simulink model "LKAS_AutoSave_DF_20211126_SW5"  (R2018b)
settings: Solver=FixedStepDiscrete  StartTime=0.0  StopTime=10.0  FixedStep=0.01  RelTol=1e-3
undefined symbols (not defined in the file): LKA_CarWidth, LKA_SampleTime, LKA_StrRatio_C, LKA_Veh2CamL_C, LKA_Veh2CamW_C, LKA_WhlBaseL_C, LL_CompSWA_C, LL_CrvtPrvwT_C, LL_DesDvt_C, LL_DvtComp_C, LL_DvtPrvwT_C, LL_DvtSpdDet_vDvtSpdMin_C, LL_HdAgExT_C, LL_HdAgPrvwT_C, LL_LAccMax_C, LL_LAccRMax_C, LL_LDW_EarliestWarnLine_C, LL_LDW_LatestWarnLine_C, LL_LDWS_SUPPRESS_HEADING, LL_LFClb_TFC_FfCtlRatio_C, LL_LFClb_TFC_KdBalance_C, LL_LFClb_TFC_KdMaxSWA_C, LL_LFClb_TFC_KdV1_C, LL_LFClb_TFC_KdV2_C, LL_LFClb_TFC_KdVehSpdLwr_C, LL_LFClb_TFC_KdVehSpdUpr_C, LL_LFClb_TFC_Ki_C, LL_LFClb_TFC_KiMaxSWA_C, LL_LFClb_TFC_Kp_C, LL_LFClb_TFC_KpKlat_C, LL_LFClb_TFC_KpV1_C, LL_LFClb_TFC_KpV2_C, LL_LFClb_TFC_KpVehSpdLwr_C, LL_LFClb_TFC_KpVehSpdUpr_C, LL_LFClb_TFC_PrvwT_C, LL_LKA_EarliestWarnLine_C, LL_LKA_LatestWarnLine_C, LL_LKAExPrcs_ExitC0Dvt, LL_LKAExPrcs_ExitC0Swt, LL_LKAExPrcs_tiExitTime1, LL_LKAExPrcs_tiExitTime2, LL_LKAExPrcs_tiExitTime3, LL_LKAS_OUT_OF_CONTROL_LAT_VEL, LL_LKAS_OUT_OF_CONTROL_TTLC, LL_LKASWASyn_M0, LL_LKASWASyn_M1, LL_LKASWASyn_M2, LL_LKASWASyn_M3K, LL_LKASWASyn_SWAaddMax, LL_LKASWASyn_T2, LL_LKASWASyn_tiTrqSwaRtTime, LL_LKASWASyn_tiTrqSwaTime, LL_LKASWASyn_TrqMax, LL_LKASWASyn_TrqSwaAddSwt, LL_LKASWASyn_TrqSwaRateDiff, LL_LSpdCompT_C, LL_lStpLngth_C, LL_MAX_DELAY_EPSSTAR_TIME, LL_MAX_DRIVER_TORQUE_DISABLE, LL_MAX_DRIVER_TORQUE_ENABLE ... (+38)
libraries: simulink x137, canmsglib x10, dspstat3 x3, simulink_extras x1
(part 11 of 13)

== system LKAS_AutoSave_DF_20211126_SW5/LKAS/LL/LLOn/LL State Determination (LLStateDet)/LL State Machine Conditions (LLSMCon)/Disable Condition (DisblC)/LKA Own Condition (LKAOwnC)/LKA Own Condition Synthesis (LKAOwnCSyn) ==
  LKAOwnCSyn_stDACMode : Inport
  LKAOwnCSyn_stVehLSpdC : Inport  Port=2
  LKAOwnCSyn_stVehPosChk : Inport  Port=3
  LKAOwnCSyn_stEPSCtlEC : Inport  Port=4
  Compare To Constant : simulink/Logic and Bit Operations/Compare To Constant  relop===  const=2  OutDataTypeStr=boolean
  Compare To Constant1 : simulink/Logic and Bit Operations/Compare To Constant  relop===  const=1  OutDataTypeStr=boolean
  Compare To Constant2 : simulink/Logic and Bit Operations/Compare To Constant  relop===  const=1  OutDataTypeStr=boolean
  Compare To Constant3 : simulink/Logic and Bit Operations/Compare To Constant  relop===  const=1  OutDataTypeStr=boolean
  Logical Operator : Logic  AllPortsSameDT=off  OutDataTypeStr=boolean
  Logical Operator1 : Logic  Operator=OR  Inputs=3  AllPortsSameDT=off  OutDataTypeStr=boolean
  LKAOwnCSyn_stLKAOwnCSyn : Outport
  wires:
  Compare To Constant3/1 -> Logical Operator1/1
  LKAOwnCSyn_stVehLSpdC/1 -> Compare To Constant3/1
  Logical Operator1/1 -> Logical Operator/2
  Compare To Constant/1 -> Logical Operator/1
  Compare To Constant1/1 -> Logical Operator1/2
  Compare To Constant2/1 -> Logical Operator1/3
  LKAOwnCSyn_stEPSCtlEC/1 -> Compare To Constant2/1
  Logical Operator/1 -> LKAOwnCSyn_stLKAOwnCSyn/1
  LKAOwnCSyn_stVehPosChk/1 -> Compare To Constant1/1
  LKAOwnCSyn_stDACMode/1 -> Compare To Constant/1

== system LKAS_AutoSave_DF_20211126_SW5/LKAS/LL/LLOn/LL State Determination (LLStateDet)/LL State Machine Conditions (LLSMCon)/Disable Condition (DisblC)/LKA Own Condition (LKAOwnC)/Vehicle Lateral Speed Condition (VehLSpdC) ==
  VehLSpdC_bsTTLC : Inport
  VehLSpdC_vVehLSpdMax_C : Inport  Port=2
  Abs : Abs
  Abs1 : Abs
  Bus Selector : BusSelector  OutputSignals=vLft,vRgt
  Logical Operator : Logic  Operator=OR  AllPortsSameDT=off  OutDataTypeStr=boolean
  Relational Operator1 : RelationalOperator  OutDataTypeStr=boolean  RndMeth=Nearest
  Relational Operator2 : RelationalOperator  OutDataTypeStr=boolean  RndMeth=Nearest
  VehLSpdC_stVehLSpdC : Outport
  wires:
  Logical Operator/1 -> VehLSpdC_stVehLSpdC/1
  Relational Operator2/1 -> Logical Operator/2
  Relational Operator1/1 -> Logical Operator/1
  VehLSpdC_vVehLSpdMax_C/1 -> Relational Operator1/2, Relational Operator2/2
  Abs1/1 -> Relational Operator2/1
  Bus Selector/2 -> Abs1/1  "<vRgt>"
  Bus Selector/1 -> Abs/1  "<vLft>"
  Abs/1 -> Relational Operator1/1
  VehLSpdC_bsTTLC/1 -> Bus Selector/1

== system LKAS_AutoSave_DF_20211126_SW5/LKAS/LL/LLOn/LL State Determination (LLStateDet)/LL State Machine Conditions (LLSMCon)/Disable Condition (DisblC)/LKA Own Condition (LKAOwnC)/Vehicle Position Check (VehPosChk) ==
  VehPosChk_lLftDvt : Inport
  VehPosChk_lRgtDvt : Inport  Port=2
  VehPosChk_lAlrmLine_C : Inport  Port=3
  Logical Operator : Logic  Operator=OR  AllPortsSameDT=off  OutDataTypeStr=boolean
  Relational Operator1 : RelationalOperator  Operator=<=  OutDataTypeStr=boolean  RndMeth=Nearest
  Relational Operator2 : RelationalOperator  Operator=<=  OutDataTypeStr=boolean  RndMeth=Nearest
  VehPosChk_stVehPosChk : Outport
  wires:
  VehPosChk_lRgtDvt/1 -> Relational Operator2/1
  VehPosChk_lLftDvt/1 -> Relational Operator1/1
  Logical Operator/1 -> VehPosChk_stVehPosChk/1
  Relational Operator2/1 -> Logical Operator/2
  Relational Operator1/1 -> Logical Operator/1
  VehPosChk_lAlrmLine_C/1 -> Relational Operator2/2, Relational Operator1/2

== system LKAS_AutoSave_DF_20211126_SW5/LKAS/LL/LLOn/LL State Determination (LLStateDet)/LL State Machine Conditions (LLSMCon)/Disable Condition (DisblC)/Lane Condition (LaneC)/Lane C1 Detection (LaneC1Det) ==
  LaneWDet_facmL0C1 : Inport
  LaneWDet_facmR0C1 : Inport  Port=2
  Abs : Abs
  Add : Sum  Inputs=+-  OutDataTypeStr=single
  Compare To Constant1 : simulink/Logic and Bit Operations/Compare To Constant  relop=>  const=0.040  OutDataTypeStr=boolean
  LaneC1Det_stLaneC1DetFlg : Outport
  wires:
  Abs/1 -> Compare To Constant1/1
  Compare To Constant1/1 -> LaneC1Det_stLaneC1DetFlg/1
  Add/1 -> Abs/1
  LaneWDet_facmL0C1/1 -> Add/1
  LaneWDet_facmR0C1/1 -> Add/2

== system LKAS_AutoSave_DF_20211126_SW5/LKAS/LL/LLOn/LL State Determination (LLStateDet)/LL State Machine Conditions (LLSMCon)/Disable Condition (DisblC)/Lane Condition (LaneC)/Lane Condition Synthesis (LaneCSyn) ==
  LaneCSyn_stLaneQlECFlg : Inport
  LaneCSyn_stLaneWDetFlg : Inport  Port=2
  LaneCSyn_stLaneCrvtDetFlg : Inport  Port=3
  LaneCSyn_stLaneC1DetFlg : Inport  Port=4
  Logical Operator3 : Logic  Operator=OR  Inputs=4  AllPortsSameDT=off  OutDataTypeStr=boolean
  LaneCSyn_stLaneCSyn : Outport
  wires:
  LaneCSyn_stLaneC1DetFlg/1 -> Logical Operator3/4
  LaneCSyn_stLaneWDetFlg/1 -> Logical Operator3/2
  Logical Operator3/1 -> LaneCSyn_stLaneCSyn/1
  LaneCSyn_stLaneCrvtDetFlg/1 -> Logical Operator3/3
  LaneCSyn_stLaneQlECFlg/1 -> Logical Operator3/1

== system LKAS_AutoSave_DF_20211126_SW5/LKAS/LL/LLOn/LL State Determination (LLStateDet)/LL State Machine Conditions (LLSMCon)/Disable Condition (DisblC)/Lane Condition (LaneC)/Lane Curvature Detection (LaneCrvtDet) ==
  LaneCrvtDet_crPrvwCrvt : Inport
  LaneCrvtDet_crLaneCrvtMax_C : Inport  Port=2
  Abs : Abs
  Constant : Constant  Value=0  OutDataTypeStr=single  SampleTime=-1
  Interval Test Dynamic : simulink/Logic and Bit Operations/Interval Test Dynamic  IntervalClosedRight=on  IntervalClosedLeft=on  OutDataTypeStr=boolean
      settings: SourceProductName=Simulink  SourceProductBaseCode=SL
  Logical Operator : Logic  Operator=NOT  AllPortsSameDT=off  OutDataTypeStr=boolean
  LaneCrvtDet_stLaneCrvtDetFlg : Outport
  wires:
  Abs/1 -> Interval Test Dynamic/2
  LaneCrvtDet_crPrvwCrvt/1 -> Abs/1
  Constant/1 -> Interval Test Dynamic/3
  LaneCrvtDet_crLaneCrvtMax_C/1 -> Interval Test Dynamic/1
  Logical Operator/1 -> LaneCrvtDet_stLaneCrvtDetFlg/1
  Interval Test Dynamic/1 -> Logical Operator/1

== system LKAS_AutoSave_DF_20211126_SW5/LKAS/LL/LLOn/LL State Determination (LLStateDet)/LL State Machine Conditions (LLSMCon)/Disable Condition (DisblC)/Lane Condition (LaneC)/Lane Quality Disable Condition (LaneQlDC) ==
  LaneQlDC_stFacmL0Ql : Inport
  LaneQlDC_stFacmR0Ql : Inport  Port=2
  Compare To Constant : simulink/Logic and Bit Operations/Compare To Constant  relop=<  const=3  OutDataTypeStr=boolean
  Compare To Constant1 : simulink/Logic and Bit Operations/Compare To Constant  relop=<  const=3  OutDataTypeStr=boolean
  Logical Operator : Logic  AllPortsSameDT=off  OutDataTypeStr=boolean
  LaneQlDC_stLaneQlDCFlg : Outport
  wires:
  Logical Operator/1 -> LaneQlDC_stLaneQlDCFlg/1
  Compare To Constant1/1 -> Logical Operator/2
  Compare To Constant/1 -> Logical Operator/1
  LaneQlDC_stFacmR0Ql/1 -> Compare To Constant1/1
  LaneQlDC_stFacmL0Ql/1 -> Compare To Constant/1

== system LKAS_AutoSave_DF_20211126_SW5/LKAS/LL/LLOn/LL State Determination (LLStateDet)/LL State Machine Conditions (LLSMCon)/Disable Condition (DisblC)/Lane Condition (LaneC)/Lane Width Detection (LaneWDet) ==
  LaneWDet_LaneWidth : Inport
  LaneWDet_lLaneWMax : Inport  Port=2
  LaneWDet_lLaneWMin : Inport  Port=3
  Abs1 : Abs
  Compare To Zero : simulink/Logic and Bit Operations/Compare To Zero  relop===  OutDataTypeStr=boolean
  Interval Test Dynamic : simulink/Logic and Bit Operations/Interval Test Dynamic  IntervalClosedRight=on  IntervalClosedLeft=on  OutDataTypeStr=boolean
      settings: SourceProductName=Simulink  SourceProductBaseCode=SL
  LaneWDet_stLaneWDetFlg : Outport
  wires:
  LaneWDet_LaneWidth/1 -> Abs1/1
  Abs1/1 -> Interval Test Dynamic/2
  LaneWDet_lLaneWMin/1 -> Interval Test Dynamic/3
  LaneWDet_lLaneWMax/1 -> Interval Test Dynamic/1
  Compare To Zero/1 -> LaneWDet_stLaneWDetFlg/1
  Interval Test Dynamic/1 -> Compare To Zero/1

== system LKAS_AutoSave_DF_20211126_SW5/LKAS/LL/LLOn/LL State Determination (LLStateDet)/LL State Machine Conditions (LLSMCon)/Disable Condition (DisblC)/Subsystem/Subsystem ==
  in1 : Inport
  Add : Sum
  Cast To Single : DataTypeConversion  OutDataTypeStr=uint8
  Memory : Memory  InheritSampleTime=on
  Saturation : Saturate  UpperLimit=1  LowerLimit=0
      settings: AttributesFormatString="Min = %<LowerLimit>  Max = %<UpperLimit>"
  Out1 : Outport
  wires:
  Saturation/1 -> Out1/1, Add/2
  Add/1 -> Memory/1
  Memory/1 -> Saturation/1
  in1/1 -> Cast To Single/1
  Cast To Single/1 -> Add/1

== system LKAS_AutoSave_DF_20211126_SW5/LKAS/LL/LLOn/LL State Determination (LLStateDet)/LL State Machine Conditions (LLSMCon)/Disable Condition (DisblC)/Subsystem/Subsystem1 ==
  in1 : Inport
  Add : Sum
  Cast To Single : DataTypeConversion  OutDataTypeStr=uint8
  Memory : Memory  InheritSampleTime=on
  Saturation : Saturate  UpperLimit=1  LowerLimit=0
      settings: AttributesFormatString="Min = %<LowerLimit>  Max = %<UpperLimit>"
  Out1 : Outport
  wires:
  Cast To Single/1 -> Add/1
  in1/1 -> Cast To Single/1
  Memory/1 -> Saturation/1
  Add/1 -> Memory/1
  Saturation/1 -> Add/2, Out1/1

== system LKAS_AutoSave_DF_20211126_SW5/LKAS/LL/LLOn/LL State Determination (LLStateDet)/LL State Machine Conditions (LLSMCon)/Disable Condition (DisblC)/Subsystem/Subsystem10 ==
  in1 : Inport
  Add : Sum
  Cast To Single : DataTypeConversion  OutDataTypeStr=uint8
  Memory : Memory  InheritSampleTime=on
  Saturation : Saturate  UpperLimit=1  LowerLimit=0
      settings: AttributesFormatString="Min = %<LowerLimit>  Max = %<UpperLimit>"
  Out1 : Outport
  wires:
  Saturation/1 -> Out1/1, Add/2
  Add/1 -> Memory/1
  Memory/1 -> Saturation/1
  in1/1 -> Cast To Single/1
  Cast To Single/1 -> Add/1

== system LKAS_AutoSave_DF_20211126_SW5/LKAS/LL/LLOn/LL State Determination (LLStateDet)/LL State Machine Conditions (LLSMCon)/Disable Condition (DisblC)/Subsystem/Subsystem11 ==
  in1 : Inport
  Add : Sum
  Cast To Single : DataTypeConversion  OutDataTypeStr=uint8
  Memory : Memory  InheritSampleTime=on
  Saturation : Saturate  UpperLimit=1  LowerLimit=0
      settings: AttributesFormatString="Min = %<LowerLimit>  Max = %<UpperLimit>"
  Out1 : Outport
  wires:
  Cast To Single/1 -> Add/1
  in1/1 -> Cast To Single/1
  Memory/1 -> Saturation/1
  Add/1 -> Memory/1
  Saturation/1 -> Add/2, Out1/1

== system LKAS_AutoSave_DF_20211126_SW5/LKAS/LL/LLOn/LL State Determination (LLStateDet)/LL State Machine Conditions (LLSMCon)/Disable Condition (DisblC)/Subsystem/Subsystem12 ==
  in1 : Inport
  Add : Sum
  Cast To Single : DataTypeConversion  OutDataTypeStr=uint8
  Memory : Memory  InheritSampleTime=on
  Saturation : Saturate  UpperLimit=1  LowerLimit=0
      settings: AttributesFormatString="Min = %<LowerLimit>  Max = %<UpperLimit>"
  Out1 : Outport
  wires:
  Saturation/1 -> Out1/1, Add/2
  Add/1 -> Memory/1
  Memory/1 -> Saturation/1
  in1/1 -> Cast To Single/1
  Cast To Single/1 -> Add/1

== system LKAS_AutoSave_DF_20211126_SW5/LKAS/LL/LLOn/LL State Determination (LLStateDet)/LL State Machine Conditions (LLSMCon)/Disable Condition (DisblC)/Subsystem/Subsystem13 ==
  in1 : Inport
  Add : Sum
  Cast To Single : DataTypeConversion  OutDataTypeStr=uint8
  Memory : Memory  InheritSampleTime=on
  Saturation : Saturate  UpperLimit=1  LowerLimit=0
      settings: AttributesFormatString="Min = %<LowerLimit>  Max = %<UpperLimit>"
  Out1 : Outport
  wires:
  Cast To Single/1 -> Add/1
  in1/1 -> Cast To Single/1
  Memory/1 -> Saturation/1
  Add/1 -> Memory/1
  Saturation/1 -> Add/2, Out1/1

== system LKAS_AutoSave_DF_20211126_SW5/LKAS/LL/LLOn/LL State Determination (LLStateDet)/LL State Machine Conditions (LLSMCon)/Disable Condition (DisblC)/Subsystem/Subsystem14 ==
  in1 : Inport
  Add : Sum
  Cast To Single : DataTypeConversion  OutDataTypeStr=uint8
  Memory : Memory  InheritSampleTime=on
  Saturation : Saturate  UpperLimit=1  LowerLimit=0
      settings: AttributesFormatString="Min = %<LowerLimit>  Max = %<UpperLimit>"
  Out1 : Outport
  wires:
  Cast To Single/1 -> Add/1
  in1/1 -> Cast To Single/1
  Memory/1 -> Saturation/1
  Add/1 -> Memory/1
  Saturation/1 -> Add/2, Out1/1

== system LKAS_AutoSave_DF_20211126_SW5/LKAS/LL/LLOn/LL State Determination (LLStateDet)/LL State Machine Conditions (LLSMCon)/Disable Condition (DisblC)/Subsystem/Subsystem15 ==
  in1 : Inport
  Add : Sum
  Cast To Single : DataTypeConversion  OutDataTypeStr=uint8
  Memory : Memory  InheritSampleTime=on
  Saturation : Saturate  UpperLimit=1  LowerLimit=0
      settings: AttributesFormatString="Min = %<LowerLimit>  Max = %<UpperLimit>"
  Out1 : Outport
  wires:
  Saturation/1 -> Out1/1, Add/2
  Add/1 -> Memory/1
  Memory/1 -> Saturation/1
  in1/1 -> Cast To Single/1
  Cast To Single/1 -> Add/1

== system LKAS_AutoSave_DF_20211126_SW5/LKAS/LL/LLOn/LL State Determination (LLStateDet)/LL State Machine Conditions (LLSMCon)/Disable Condition (DisblC)/Subsystem/Subsystem16 ==
  in1 : Inport
  Add : Sum
  Cast To Single : DataTypeConversion  OutDataTypeStr=uint8
  Memory : Memory  InheritSampleTime=on
  Saturation : Saturate  UpperLimit=1  LowerLimit=0
      settings: AttributesFormatString="Min = %<LowerLimit>  Max = %<UpperLimit>"
  Out1 : Outport
  wires:
  Saturation/1 -> Out1/1, Add/2
  Add/1 -> Memory/1
  Memory/1 -> Saturation/1
  in1/1 -> Cast To Single/1
  Cast To Single/1 -> Add/1

== system LKAS_AutoSave_DF_20211126_SW5/LKAS/LL/LLOn/LL State Determination (LLStateDet)/LL State Machine Conditions (LLSMCon)/Disable Condition (DisblC)/Subsystem/Subsystem17 ==
  in1 : Inport
  Add : Sum
  Cast To Single : DataTypeConversion  OutDataTypeStr=uint8
  Memory : Memory  InheritSampleTime=on
  Saturation : Saturate  UpperLimit=1  LowerLimit=0
      settings: AttributesFormatString="Min = %<LowerLimit>  Max = %<UpperLimit>"
  Out1 : Outport
  wires:
  Cast To Single/1 -> Add/1
  in1/1 -> Cast To Single/1
  Memory/1 -> Saturation/1
  Add/1 -> Memory/1
  Saturation/1 -> Add/2, Out1/1

== system LKAS_AutoSave_DF_20211126_SW5/LKAS/LL/LLOn/LL State Determination (LLStateDet)/LL State Machine Conditions (LLSMCon)/Disable Condition (DisblC)/Subsystem/Subsystem2 ==
  in1 : Inport
  Add : Sum
  Cast To Single : DataTypeConversion  OutDataTypeStr=uint8
  Memory : Memory  InheritSampleTime=on
  Saturation : Saturate  UpperLimit=1  LowerLimit=0
      settings: AttributesFormatString="Min = %<LowerLimit>  Max = %<UpperLimit>"
  Out1 : Outport
  wires:
  Cast To Single/1 -> Add/1
  in1/1 -> Cast To Single/1
  Memory/1 -> Saturation/1
  Add/1 -> Memory/1
  Saturation/1 -> Add/2, Out1/1

== system LKAS_AutoSave_DF_20211126_SW5/LKAS/LL/LLOn/LL State Determination (LLStateDet)/LL State Machine Conditions (LLSMCon)/Disable Condition (DisblC)/Subsystem/Subsystem3 ==
  in1 : Inport
  Add : Sum
  Cast To Single : DataTypeConversion  OutDataTypeStr=uint8
  Memory : Memory  InheritSampleTime=on
  Saturation : Saturate  UpperLimit=1  LowerLimit=0
      settings: AttributesFormatString="Min = %<LowerLimit>  Max = %<UpperLimit>"
  Out1 : Outport
  wires:
  Saturation/1 -> Out1/1, Add/2
  Add/1 -> Memory/1
  Memory/1 -> Saturation/1
  in1/1 -> Cast To Single/1
  Cast To Single/1 -> Add/1

== system LKAS_AutoSave_DF_20211126_SW5/LKAS/LL/LLOn/LL State Determination (LLStateDet)/LL State Machine Conditions (LLSMCon)/Disable Condition (DisblC)/Subsystem/Subsystem4 ==
  in1 : Inport
  Add : Sum
  Cast To Single : DataTypeConversion  OutDataTypeStr=uint8
  Memory : Memory  InheritSampleTime=on
  Saturation : Saturate  UpperLimit=1  LowerLimit=0
      settings: AttributesFormatString="Min = %<LowerLimit>  Max = %<UpperLimit>"
  Out1 : Outport
  wires:
  Cast To Single/1 -> Add/1
  in1/1 -> Cast To Single/1
  Memory/1 -> Saturation/1
  Add/1 -> Memory/1
  Saturation/1 -> Add/2, Out1/1

== system LKAS_AutoSave_DF_20211126_SW5/LKAS/LL/LLOn/LL State Determination (LLStateDet)/LL State Machine Conditions (LLSMCon)/Disable Condition (DisblC)/Subsystem/Subsystem5 ==
  in1 : Inport
  Add : Sum
  Cast To Single : DataTypeConversion  OutDataTypeStr=uint8
  Memory : Memory  InheritSampleTime=on
  Saturation : Saturate  UpperLimit=1  LowerLimit=0
      settings: AttributesFormatString="Min = %<LowerLimit>  Max = %<UpperLimit>"
  Out1 : Outport
  wires:
  Saturation/1 -> Out1/1, Add/2
  Add/1 -> Memory/1
  Memory/1 -> Saturation/1
  in1/1 -> Cast To Single/1
  Cast To Single/1 -> Add/1

== system LKAS_AutoSave_DF_20211126_SW5/LKAS/LL/LLOn/LL State Determination (LLStateDet)/LL State Machine Conditions (LLSMCon)/Disable Condition (DisblC)/Subsystem/Subsystem6 ==
  in1 : Inport
  Add : Sum
  Cast To Single : DataTypeConversion  OutDataTypeStr=uint8
  Memory : Memory  InheritSampleTime=on
  Saturation : Saturate  UpperLimit=1  LowerLimit=0
      settings: AttributesFormatString="Min = %<LowerLimit>  Max = %<UpperLimit>"
  Out1 : Outport
  wires:
  Saturation/1 -> Out1/1, Add/2
  Add/1 -> Memory/1
  Memory/1 -> Saturation/1
  in1/1 -> Cast To Single/1
  Cast To Single/1 -> Add/1

== system LKAS_AutoSave_DF_20211126_SW5/LKAS/LL/LLOn/LL State Determination (LLStateDet)/LL State Machine Conditions (LLSMCon)/Disable Condition (DisblC)/Subsystem/Subsystem7 ==
  in1 : Inport
  Add : Sum
  Cast To Single : DataTypeConversion  OutDataTypeStr=uint8
  Memory : Memory  InheritSampleTime=on
  Saturation : Saturate  UpperLimit=1  LowerLimit=0
      settings: AttributesFormatString="Min = %<LowerLimit>  Max = %<UpperLimit>"
  Out1 : Outport
  wires:
  Cast To Single/1 -> Add/1
  in1/1 -> Cast To Single/1
  Memory/1 -> Saturation/1
  Add/1 -> Memory/1
  Saturation/1 -> Add/2, Out1/1

== system LKAS_AutoSave_DF_20211126_SW5/LKAS/LL/LLOn/LL State Determination (LLStateDet)/LL State Machine Conditions (LLSMCon)/Disable Condition (DisblC)/Subsystem/Subsystem8 ==
  in1 : Inport
  Add : Sum
  Cast To Single : DataTypeConversion  OutDataTypeStr=uint8
  Memory : Memory  InheritSampleTime=on
  Saturation : Saturate  UpperLimit=1  LowerLimit=0
      settings: AttributesFormatString="Min = %<LowerLimit>  Max = %<UpperLimit>"
  Out1 : Outport
  wires:
  Cast To Single/1 -> Add/1
  in1/1 -> Cast To Single/1
  Memory/1 -> Saturation/1
  Add/1 -> Memory/1
  Saturation/1 -> Add/2, Out1/1

== system LKAS_AutoSave_DF_20211126_SW5/LKAS/LL/LLOn/LL State Determination (LLStateDet)/LL State Machine Conditions (LLSMCon)/Disable Condition (DisblC)/Subsystem/Subsystem9 ==
  in1 : Inport
  Add : Sum
  Cast To Single : DataTypeConversion  OutDataTypeStr=uint8
  Memory : Memory  InheritSampleTime=on
  Saturation : Saturate  UpperLimit=1  LowerLimit=0
      settings: AttributesFormatString="Min = %<LowerLimit>  Max = %<UpperLimit>"
  Out1 : Outport
  wires:
  Saturation/1 -> Out1/1, Add/2
  Add/1 -> Memory/1
  Memory/1 -> Saturation/1
  in1/1 -> Cast To Single/1
  Cast To Single/1 -> Add/1

== system LKAS_AutoSave_DF_20211126_SW5/LKAS/LL/LLOn/LL State Determination (LLStateDet)/LL State Machine Conditions (LLSMCon)/Disable Condition (DisblC)/Vehicle State Condition (VehStateC)/Emergency Light Enable Condition (EmgcyLghtEC) ==
  EmgcyLghtEC_bsStLampState : Inport
  Add : Sum
  Bus Selector : BusSelector  OutputSignals=BCM_Double_Light,BCM_Left_Light,BCM_Right_Light
  Compare To Constant : simulink/Logic and Bit Operations/Compare To Constant  relop=>  const=1  OutDataTypeStr=boolean
  Compare To Constant1 : simulink/Logic and Bit Operations/Compare To Constant  relop=>  const=0  OutDataTypeStr=boolean
  Compare To Constant2 : simulink/Logic and Bit Operations/Compare To Constant  relop=>  const=0  OutDataTypeStr=boolean
  Compare To Constant3 : simulink/Logic and Bit Operations/Compare To Constant  relop=>  const=0  OutDataTypeStr=boolean
  Constant : Constant  Value=3  OutDataTypeStr=single
  Constant1 : Constant  Value=-1  OutDataTypeStr=single
  Logical Operator : Logic  Operator=OR  Inputs=3  AllPortsSameDT=off  OutDataTypeStr=boolean
  Memory : Memory  InheritSampleTime=on
  Saturation : Saturate  UpperLimit=200  LowerLimit=-1
      settings: AttributesFormatString="Min = %<LowerLimit>  Max = %<UpperLimit>"
  Switch : Switch  Criteria=u2 > Threshold
  EmgcyLghtEC_stEmgcyLghtECFlg : Outport
  wires:
  Compare To Constant3/1 -> Logical Operator/3
  Bus Selector/3 -> Compare To Constant3/1  "<BCM_Right_Light>"
  Compare To Constant/1 -> EmgcyLghtEC_stEmgcyLghtECFlg/1
  Memory/1 -> Add/2
  Saturation/1 -> Memory/1, Compare To Constant/1
  Add/1 -> Saturation/1
  Switch/1 -> Add/1
  Constant1/1 -> Switch/3
  Constant/1 -> Switch/1
  Logical Operator/1 -> Switch/2
  Bus Selector/2 -> Compare To Constant2/1  "<BCM_Left_Light>"
  Bus Selector/1 -> Compare To Constant1/1  "<BCM_Double_Light>"
  EmgcyLghtEC_bsStLampState/1 -> Bus Selector/1
  Compare To Constant1/1 -> Logical Operator/1
  Compare To Constant2/1 -> Logical Operator/2

== system LKAS_AutoSave_DF_20211126_SW5/LKAS/LL/LLOn/LL State Determination (LLStateDet)/LL State Machine Conditions (LLSMCon)/Disable Condition (DisblC)/Vehicle State Condition (VehStateC)/Gear Disable Condition (GearDC) ==
  In1 : Inport
  Compare To Constant : simulink/Logic and Bit Operations/Compare To Constant  relop=~=  const=3  OutDataTypeStr=boolean
  GearDC_stGearDCFlg : Outport
  wires:
  Compare To Constant/1 -> GearDC_stGearDCFlg/1
  In1/1 -> Compare To Constant/1

== system LKAS_AutoSave_DF_20211126_SW5/LKAS/LL/LLOn/LL State Determination (LLStateDet)/LL State Machine Conditions (LLSMCon)/Disable Condition (DisblC)/Vehicle State Condition (VehStateC)/Vehicle Speed Disable Condition (VehSpdDC) ==
  VehSpdDC_stDACMode : Inport
  VehSpdDC_vVehSpd : Inport  Port=2
  VehSpdDC_vLDWVehSpdMax_C : Inport  Port=3
  VehSpdDC_vLKAVehSpdMax_C : Inport  Port=4
  VehSpdDC_vVehSpdMin_C : Inport  Port=5
  Interval Test Dynamic : simulink/Logic and Bit Operations/Interval Test Dynamic  IntervalClosedRight=off  IntervalClosedLeft=off  OutDataTypeStr=boolean
      settings: SourceProductName=Simulink  SourceProductBaseCode=SL
  Logical Operator : Logic  Operator=NOT  AllPortsSameDT=off  OutDataTypeStr=boolean
  Switch : Switch  Threshold=2
  VehSpdDC_stVehSpdDCFlg : Outport
  wires:
  VehSpdDC_vLDWVehSpdMax_C/1 -> Switch/3
  Switch/1 -> Interval Test Dynamic/1
  VehSpdDC_vLKAVehSpdMax_C/1 -> Switch/1
  VehSpdDC_stDACMode/1 -> Switch/2
  Logical Operator/1 -> VehSpdDC_stVehSpdDCFlg/1
  VehSpdDC_vVehSpdMin_C/1 -> Interval Test Dynamic/3
  VehSpdDC_vVehSpd/1 -> Interval Test Dynamic/2
  Interval Test Dynamic/1 -> Logical Operator/1

== system LKAS_AutoSave_DF_20211126_SW5/LKAS/LL/LLOn/LL State Determination (LLStateDet)/LL State Machine Conditions (LLSMCon)/Disable Condition (DisblC)/Vehicle State Condition (VehStateC)/Vehicle State Condition Synthesis (VehStateCSyn) ==
  VehStateCSyn_stVehSpdDCFlg : Inport
  VehStateCSyn_stEmgcyLghtDCFlg : Inport  Port=2
  VehStateCSyn_stGearDCFlg : Inport  Port=3
  Logical Operator3 : Logic  Operator=OR  Inputs=3  AllPortsSameDT=off  OutDataTypeStr=boolean
  VehStateCSyn_stVehStateCSyn : Outport
  wires:
  VehStateCSyn_stEmgcyLghtDCFlg/1 -> Logical Operator3/2
  Logical Operator3/1 -> VehStateCSyn_stVehStateCSyn/1
  VehStateCSyn_stGearDCFlg/1 -> Logical Operator3/3
  VehStateCSyn_stVehSpdDCFlg/1 -> Logical Operator3/1

== system LKAS_AutoSave_DF_20211126_SW5/LKAS/LL/LLOn/LL State Determination (LLStateDet)/LL State Machine Conditions (LLSMCon)/Enable Condition (EnaC)/Enable Condition Synthesis (EnaCSyn)/If Action Subsystem ==
  Action Port : ActionPort  InitializeStates=reset  ActionType=then
      settings: AttributesFormatString=states = %<InitializeStates>
  Constant : Constant  OutDataTypeStr=boolean  SampleTime=-1
  Out : Outport
      settings: AttributesFormatString=%<OutputWhenDisabled> = %<InitialOutput>
  wires:
  Constant/1 -> Out/1

== system LKAS_AutoSave_DF_20211126_SW5/LKAS/LL/LLOn/LL State Determination (LLStateDet)/LL State Machine Conditions (LLSMCon)/Enable Condition (EnaC)/Enable Condition Synthesis (EnaCSyn)/If Action Subsystem2 ==
  Action Port : ActionPort  InitializeStates=reset  ActionType=then
      settings: AttributesFormatString=states = %<InitializeStates>
  Constant : Constant  OutDataTypeStr=boolean  SampleTime=-1
  Out : Outport
      settings: AttributesFormatString=%<OutputWhenDisabled> = %<InitialOutput>
  wires:
  Constant/1 -> Out/1

== system LKAS_AutoSave_DF_20211126_SW5/LKAS/LL/LLOn/LL State Determination (LLStateDet)/LL State Machine Conditions (LLSMCon)/Enable Condition (EnaC)/Enable Condition Synthesis (EnaCSyn)/If Action Subsystem3 ==
  Action Port : ActionPort  InitializeStates=reset  ActionType=else
      settings: AttributesFormatString=states = %<InitializeStates>
  Constant : Constant  Value=0  OutDataTypeStr=boolean
  Out : Outport
      settings: AttributesFormatString=%<OutputWhenDisabled> = %<InitialOutput>
  wires:
  Constant/1 -> Out/1

== system LKAS_AutoSave_DF_20211126_SW5/LKAS/LL/LLOn/LL State Determination (LLStateDet)/LL State Machine Conditions (LLSMCon)/Enable Condition (EnaC)/Enable Condition Synthesis (EnaCSyn)/If Action Subsystem4 ==
  Action Port : ActionPort  InitializeStates=reset  ActionType=else
      settings: AttributesFormatString=states = %<InitializeStates>
  Constant : Constant  Value=0  OutDataTypeStr=boolean
  Out : Outport
      settings: AttributesFormatString=%<OutputWhenDisabled> = %<InitialOutput>
  wires:
  Constant/1 -> Out/1

== system LKAS_AutoSave_DF_20211126_SW5/LKAS/LL/LLOn/LL State Determination (LLStateDet)/LL State Machine Conditions (LLSMCon)/Enable Condition (EnaC)/LDW Own Condition (LDWOwnC)/LDW Own Condition Synthesis (LDWOwnCSyn) ==
  LDWOwnCSyn_stDACMode : Inport
  LDWOwnCSyn_stVehPosChk : Inport  Port=2
  Compare To Constant : simulink/Logic and Bit Operations/Compare To Constant  relop=>=  const=1  OutDataTypeStr=boolean
  Compare To Constant1 : simulink/Logic and Bit Operations/Compare To Constant  relop===  const=1  OutDataTypeStr=boolean
  Logical Operator : Logic  AllPortsSameDT=off  OutDataTypeStr=boolean
  LDWOwnCSyn_stLDWOwnCSyn : Outport
  wires:
  Logical Operator/1 -> LDWOwnCSyn_stLDWOwnCSyn/1
  Compare To Constant1/1 -> Logical Operator/2
  Compare To Constant/1 -> Logical Operator/1
  LDWOwnCSyn_stVehPosChk/1 -> Compare To Constant1/1
  LDWOwnCSyn_stDACMode/1 -> Compare To Constant/1

== system LKAS_AutoSave_DF_20211126_SW5/LKAS/LL/LLOn/LL State Determination (LLStateDet)/LL State Machine Conditions (LLSMCon)/Enable Condition (EnaC)/LDW Own Condition (LDWOwnC)/Vehicle Position Check (VehPosChk) ==
  VehPosChk_LaneWidth : Inport
  VehPosChk_bsDvtInfo : Inport  Port=2
  VehPosChk_lWarnLine_C : Inport  Port=3
  VehPosChk_CarWidth : Inport  Port=4
  Bus Selector : BusSelector  OutputSignals=ILftDvt,IRgtDvt
  Logical Operator : Logic  AllPortsSameDT=off  OutDataTypeStr=boolean
  Relational Operator1 : RelationalOperator  OutDataTypeStr=boolean  RndMeth=Nearest
  Relational Operator2 : RelationalOperator  OutDataTypeStr=boolean  RndMeth=Nearest
  Subsystem : Subsystem
  VehPosChk_stVehPosChk : Outport
  wires:
  VehPosChk_CarWidth/1 -> Subsystem/3(CarWidth)
  VehPosChk_LaneWidth/1 -> Subsystem/2(LaneWidth)
  VehPosChk_lWarnLine_C/1 -> Subsystem/1(WarnLine_C)
  Subsystem/1(EnableLine) -> Relational Operator2/2, Relational Operator1/2
  VehPosChk_bsDvtInfo/1 -> Bus Selector/1
  Logical Operator/1 -> VehPosChk_stVehPosChk/1
  Relational Operator2/1 -> Logical Operator/2
  Relational Operator1/1 -> Logical Operator/1
  Bus Selector/2 -> Relational Operator2/1  "<IRgtDvt>"
  Bus Selector/1 -> Relational Operator1/1  "<ILftDvt>"

== system LKAS_AutoSave_DF_20211126_SW5/LKAS/LL/LLOn/LL State Determination (LLStateDet)/LL State Machine Conditions (LLSMCon)/Enable Condition (EnaC)/LKA Own Condition (LKAOwnC)/EPS State Condition (EPSStC) ==
  EPSStC_bsEPSInfo : Inport
  Bus Selector : BusSelector  OutputSignals=EPS_LKA_State
  Compare To Constant1 : simulink/Logic and Bit Operations/Compare To Constant  relop===  const=2  OutDataTypeStr=boolean
  Compare To Constant2 : simulink/Logic and Bit Operations/Compare To Constant  relop===  const=1  OutDataTypeStr=boolean
  Logical Operator : Logic  Operator=OR  AllPortsSameDT=off  OutDataTypeStr=boolean
  EPSStC_tfEPSCtlEC : Outport
  wires:
  Compare To Constant2/1 -> Logical Operator/2
  Compare To Constant1/1 -> Logical Operator/1
  Bus Selector/1 -> Compare To Constant1/1, Compare To Constant2/1  "<EPS_LKA_State>"
  Logical Operator/1 -> EPSStC_tfEPSCtlEC/1
  EPSStC_bsEPSInfo/1 -> Bus Selector/1

== system LKAS_AutoSave_DF_20211126_SW5/LKAS/LL/LLOn/LL State Determination (LLStateDet)/LL State Machine Conditions (LLSMCon)/Enable Condition (EnaC)/LKA Own Condition (LKAOwnC)/Exit Lane Delay (ExLaneDel) ==
  ExLaneDel_stVehExLane : Inport
  ExLaneDel_tiExLaneDelT : Inport  Port=2
  Bus Selector2 : BusSelector  OutputSignals=LKA_SampleTime
  Cast To Single1 : DataTypeConversion  OutDataTypeStr=uint16
  Compare To Zero : simulink/Logic and Bit Operations/Compare To Zero  relop===  OutDataTypeStr=boolean
  Detect Fall Nonpositive : simulink/Logic and Bit Operations/Detect Fall Nonpositive  vinit=0  OutDataTypeStr=boolean
      settings: SourceProductName=Simulink  SourceProductBaseCode=SL
  Detect Rise Positive1 : simulink/Logic and Bit Operations/Detect Rise Positive  vinit=0  OutDataTypeStr=boolean
  Divide : Product  Inputs=*/
  If Action Subsystem3 : Subsystem  TreatAsAtomicUnit=on
  If Action Subsystem4 : Subsystem  TreatAsAtomicUnit=on
  If Action Subsystem5 : Subsystem  TreatAsAtomicUnit=on
  If1 : If  NumInputs=4  IfExpression=u1 == 1 & u2 == 1  ElseIfExpressions=u3 == 0 & u4 == 1
  Memory1 : Memory  InheritSampleTime=on
  Memory2 : Memory  InheritSampleTime=on
  Merge : Merge  Inputs=3
  Sum Condition1 : Subsystem  TreatAsAtomicUnit=on
  ExLaneDel_stExLaneDel : Outport
  wires:
  Cast To Single1/1 -> Sum Condition1/2(Sum)
  [LLClb_bsConstantClb] -> Bus Selector2/1
  Bus Selector2/1 -> Divide/2  "<LKA_SampleTime>"
  Divide/1 -> Cast To Single1/1
  Compare To Zero/1 -> ExLaneDel_stExLaneDel/1
  Sum Condition1/1(Out) -> Memory2/1
  If Action Subsystem4/1(Out) -> Merge/2
  If Action Subsystem5/1(Out) -> Merge/3
  If Action Subsystem3/1(Out) -> Merge/1
  Detect Fall Nonpositive/1 -> If1/4
  ExLaneDel_stVehExLane/1 -> Detect Rise Positive1/1, If1/1
  Detect Rise Positive1/1 -> If1/2
  If1/3 -> If Action Subsystem5/Action
  If1/1 -> If Action Subsystem3/Action
  If1/2 -> If Action Subsystem4/Action
  ExLaneDel_tiExLaneDelT/1 -> Divide/1
  Memory2/1 -> If1/3, Detect Fall Nonpositive/1
  Memory1/1 -> If Action Subsystem5/1(In1)
  Merge/1 -> Compare To Zero/1, Sum Condition1/Enable, Sum Condition1/1(In), Memory1/1

== system LKAS_AutoSave_DF_20211126_SW5/LKAS/LL/LLOn/LL State Determination (LLStateDet)/LL State Machine Conditions (LLSMCon)/Enable Condition (EnaC)/LKA Own Condition (LKAOwnC)/LKA Own Condition Synthesis (LKAOwnCSyn) ==
  LKAOwnCSyn_stDACMode : Inport
  LKAOwnCSyn_stEPSCtlEC : Inport  Port=2
  LKAOwnCSyn_stVehLSpdC : Inport  Port=3
  LKAOwnCSyn_stVehPosChk : Inport  Port=4
  LKAOwnCSyn_stExLaneDel : Inport  Port=5
  Compare To Constant : simulink/Logic and Bit Operations/Compare To Constant  relop===  const=2  OutDataTypeStr=boolean
  Compare To Constant{1..2,4..5} (4 alike) : simulink/Logic and Bit Operations/Compare To Constant  relop===  const=1  OutDataTypeStr=boolean
  Logical Operator : Logic  Inputs=4  AllPortsSameDT=off  OutDataTypeStr=boolean
  LKAOwnCSyn_stLKAPptyCSyn : Outport
  wires:
  LKAOwnCSyn_stVehLSpdC/1 -> Compare To Constant4/1
  Compare To Constant5/1 -> ?
  Compare To Constant1/1 -> Logical Operator/4
  Compare To Constant4/1 -> Logical Operator/3
  Compare To Constant2/1 -> Logical Operator/2
  Compare To Constant/1 -> Logical Operator/1
  LKAOwnCSyn_stExLaneDel/1 -> Compare To Constant5/1
  LKAOwnCSyn_stEPSCtlEC/1 -> Compare To Constant2/1
  Logical Operator/1 -> LKAOwnCSyn_stLKAPptyCSyn/1
  LKAOwnCSyn_stVehPosChk/1 -> Compare To Constant1/1
  LKAOwnCSyn_stDACMode/1 -> Compare To Constant/1

== system LKAS_AutoSave_DF_20211126_SW5/LKAS/LL/LLOn/LL State Determination (LLStateDet)/LL State Machine Conditions (LLSMCon)/Enable Condition (EnaC)/LKA Own Condition (LKAOwnC)/Vehicle Lateral Speed Condition (VehLSpdC) ==
  VehLSpdC_bsTTLCInfo : Inport
  VehLSpdC_vVehLSpdMax_C : Inport  Port=2
  Abs1 : Abs
  Abs2 : Abs
  Bus Selector2 : BusSelector  OutputSignals=vLft,vRgt
  Logical Operator : Logic  AllPortsSameDT=off  OutDataTypeStr=boolean
  Relational Operator2 : RelationalOperator  Operator=<=  OutDataTypeStr=boolean  RndMeth=Nearest
  Relational Operator3 : RelationalOperator  Operator=<=  OutDataTypeStr=boolean  RndMeth=Nearest
  VehLSpdC_stVehLSpdC : Outport
  wires:
  Relational Operator3/1 -> Logical Operator/2
  Logical Operator/1 -> VehLSpdC_stVehLSpdC/1
  VehLSpdC_bsTTLCInfo/1 -> Bus Selector2/1
  Bus Selector2/2 -> Abs2/1  "<vRgt>"
  Bus Selector2/1 -> Abs1/1  "<vLft>"
  Abs2/1 -> Relational Operator3/1
  Relational Operator2/1 -> Logical Operator/1
  Abs1/1 -> Relational Operator2/1
  VehLSpdC_vVehLSpdMax_C/1 -> Relational Operator2/2, Relational Operator3/2

== system LKAS_AutoSave_DF_20211126_SW5/LKAS/LL/LLOn/LL State Determination (LLStateDet)/LL State Machine Conditions (LLSMCon)/Enable Condition (EnaC)/LKA Own Condition (LKAOwnC)/Vehicle Position Check (VehPosChk)1 ==
  VehPosChk_LaneWidth : Inport
  VehPosChk_bsDvtInfo : Inport  Port=2
  VehPosChk_LKALineMax : Inport  Port=3
  VehPosChk_CarWidth : Inport  Port=4
  VehPosChk_lWarnLineMax_C : Inport  Port=5
  VehPosChk_lWarnLineMin_C : Inport  Port=6
  Bus Selector : BusSelector  OutputSignals=ILftDvt,IRgtDvt
  Logical Operator : Logic  AllPortsSameDT=off  OutDataTypeStr=boolean
  Logical Operator1 : Logic  Operator=OR  AllPortsSameDT=off  OutDataTypeStr=boolean
  Relational Operator1 : RelationalOperator  OutDataTypeStr=boolean  RndMeth=Nearest
  Relational Operator2 : RelationalOperator  OutDataTypeStr=boolean  RndMeth=Nearest
  Relational Operator3 : RelationalOperator  Operator=<=  OutDataTypeStr=boolean  RndMeth=Nearest
  Relational Operator4 : RelationalOperator  Operator=<=  OutDataTypeStr=boolean  RndMeth=Nearest
  Subsystem : Subsystem
  VehPosChk_stVehPosChk : Outport
  VehPosChk_stVehExLane : Outport  Port=2
  wires:
  VehPosChk_CarWidth/1 -> Subsystem/4(VehPosChk_CarWidth)
  VehPosChk_LKALineMax/1 -> Subsystem/3(VehPosChk_LKALineMax)
  Relational Operator4/1 -> Logical Operator1/1
  VehPosChk_lWarnLineMin_C/1 -> Relational Operator4/2, Relational Operator3/2
  Relational Operator3/1 -> Logical Operator1/2
  Logical Operator1/1 -> VehPosChk_stVehExLane/1
  VehPosChk_LaneWidth/1 -> Subsystem/2(LaneWidth)
  VehPosChk_lWarnLineMax_C/1 -> Subsystem/1(WarnLine_C)
  Subsystem/1(EnableLine) -> Relational Operator2/2, Relational Operator1/2
  VehPosChk_bsDvtInfo/1 -> Bus Selector/1
  Logical Operator/1 -> VehPosChk_stVehPosChk/1
  Relational Operator2/1 -> Logical Operator/2
  Relational Operator1/1 -> Logical Operator/1
  Bus Selector/2 -> Relational Operator3/1, Relational Operator2/1  "<IRgtDvt>"
  Bus Selector/1 -> Relational Operator1/1, Relational Operator4/1  "<ILftDvt>"

== system LKAS_AutoSave_DF_20211126_SW5/LKAS/LL/LLOn/LL State Determination (LLStateDet)/LL State Machine Conditions (LLSMCon)/Enable Condition (EnaC)/Lane Condition (LaneC)/Lane C1 Detection (LaneC1Det) ==
  LaneWDet_facmL0C1 : Inport
  LaneWDet_facmR0C1 : Inport  Port=2
  Abs : Abs
  Add : Sum  Inputs=+-  OutDataTypeStr=single
  Compare To Constant1 : simulink/Logic and Bit Operations/Compare To Constant  relop=<=  const=0.025  OutDataTypeStr=boolean
  LaneC1Det_stLaneC1DetFlg : Outport
  wires:
  Abs/1 -> Compare To Constant1/1
  Compare To Constant1/1 -> LaneC1Det_stLaneC1DetFlg/1
  Add/1 -> Abs/1
  LaneWDet_facmL0C1/1 -> Add/1
  LaneWDet_facmR0C1/1 -> Add/2

== system LKAS_AutoSave_DF_20211126_SW5/LKAS/LL/LLOn/LL State Determination (LLStateDet)/LL State Machine Conditions (LLSMCon)/Enable Condition (EnaC)/Lane Condition (LaneC)/Lane Condition Synthesis (LaneCSyn) ==
  LaneCSyn_stLaneQlECFlg : Inport
  LaneCSyn_stLaneWDetFlg : Inport  Port=2
  LaneCSyn_stLaneCrvtDetFlg : Inport  Port=3
  LaneCSyn_stLaneC1DetFlg : Inport  Port=4
  Logical Operator3 : Logic  Inputs=4  AllPortsSameDT=off  OutDataTypeStr=boolean
  LaneCSyn_stLaneCSyn : Outport
  wires:
  LaneCSyn_stLaneC1DetFlg/1 -> Logical Operator3/4
  LaneCSyn_stLaneWDetFlg/1 -> Logical Operator3/2
  Logical Operator3/1 -> LaneCSyn_stLaneCSyn/1
  LaneCSyn_stLaneCrvtDetFlg/1 -> Logical Operator3/3
  LaneCSyn_stLaneQlECFlg/1 -> Logical Operator3/1

== system LKAS_AutoSave_DF_20211126_SW5/LKAS/LL/LLOn/LL State Determination (LLStateDet)/LL State Machine Conditions (LLSMCon)/Enable Condition (EnaC)/Lane Condition (LaneC)/Lane Curvature Detection (LaneCrvtDet) ==
  LaneCrvtDet_crPrvwCrvt : Inport
  LaneCrvtDet_crLaneCrvtMax_C : Inport  Port=2
  Abs : Abs
  Constant : Constant  Value=0  OutDataTypeStr=single  SampleTime=-1
  Interval Test Dynamic : simulink/Logic and Bit Operations/Interval Test Dynamic  IntervalClosedRight=on  IntervalClosedLeft=on  OutDataTypeStr=boolean
      settings: SourceProductName=Simulink  SourceProductBaseCode=SL
  LaneCrvtDet_stLaneCrvtDetFlg : Outport
  wires:
  Abs/1 -> Interval Test Dynamic/2
  LaneCrvtDet_crPrvwCrvt/1 -> Abs/1
  Constant/1 -> Interval Test Dynamic/3
  LaneCrvtDet_crLaneCrvtMax_C/1 -> Interval Test Dynamic/1
  Interval Test Dynamic/1 -> LaneCrvtDet_stLaneCrvtDetFlg/1

== system LKAS_AutoSave_DF_20211126_SW5/LKAS/LL/LLOn/LL State Determination (LLStateDet)/LL State Machine Conditions (LLSMCon)/Enable Condition (EnaC)/Lane Condition (LaneC)/Lane Quality Enable Condition (LaneQlEC) ==
  LaneQlEC_stFacmL0Ql : Inport
  LaneQlEC_stFacmR0Ql : Inport  Port=2
  Compare To Constant : simulink/Logic and Bit Operations/Compare To Constant  relop=>  const=2  OutDataTypeStr=boolean
  Compare To Constant1 : simulink/Logic and Bit Operations/Compare To Constant  relop=>  const=2  OutDataTypeStr=boolean
  Logical Operator : Logic  AllPortsSameDT=off  OutDataTypeStr=boolean
  LaneQlEC_stLaneQlECFlg : Outport
  wires:
  Logical Operator/1 -> LaneQlEC_stLaneQlECFlg/1
  Compare To Constant1/1 -> Logical Operator/2
  Compare To Constant/1 -> Logical Operator/1
  LaneQlEC_stFacmR0Ql/1 -> Compare To Constant1/1
  LaneQlEC_stFacmL0Ql/1 -> Compare To Constant/1

== system LKAS_AutoSave_DF_20211126_SW5/LKAS/LL/LLOn/LL State Determination (LLStateDet)/LL State Machine Conditions (LLSMCon)/Enable Condition (EnaC)/Lane Condition (LaneC)/Lane Width Detection (LaneWDet) ==
  LaneWDet_LaneWidth : Inport
  LaneWDet_lLaneWMax : Inport  Port=2
  LaneWDet_lLaneWMin : Inport  Port=3
  Abs1 : Abs
  Interval Test Dynamic : simulink/Logic and Bit Operations/Interval Test Dynamic  IntervalClosedRight=on  IntervalClosedLeft=on  OutDataTypeStr=boolean
      settings: SourceProductName=Simulink  SourceProductBaseCode=SL
  LaneWDet_stLaneWDetFlg : Outport
  wires:
  LaneWDet_LaneWidth/1 -> Abs1/1
  Abs1/1 -> Interval Test Dynamic/2
  LaneWDet_lLaneWMin/1 -> Interval Test Dynamic/3
  LaneWDet_lLaneWMax/1 -> Interval Test Dynamic/1
  Interval Test Dynamic/1 -> LaneWDet_stLaneWDetFlg/1

== system LKAS_AutoSave_DF_20211126_SW5/LKAS/LL/LLOn/LL State Determination (LLStateDet)/LL State Machine Conditions (LLSMCon)/Enable Condition (EnaC)/Vehicle State Condition (VehStateC)/Emergency Light Enable Condition (EmgcyLghtEC) ==
  EmgcyLghtEC_bsStLampState : Inport
  Add : Sum
  Bus Selector : BusSelector  OutputSignals=BCM_Double_Light,BCM_Left_Light,BCM_Right_Light
  Compare To Constant : simulink/Logic and Bit Operations/Compare To Constant  relop=<=  const=0  OutDataTypeStr=boolean
  Compare To Constant1 : simulink/Logic and Bit Operations/Compare To Constant  relop=>  const=0  OutDataTypeStr=boolean
  Compare To Constant2 : simulink/Logic and Bit Operations/Compare To Constant  relop=>  const=0  OutDataTypeStr=boolean
  Compare To Constant3 : simulink/Logic and Bit Operations/Compare To Constant  relop=>  const=0  OutDataTypeStr=boolean
  Constant : Constant  Value=3  OutDataTypeStr=single
  Constant1 : Constant  Value=-1  OutDataTypeStr=single
  Logical Operator : Logic  Operator=OR  Inputs=3  AllPortsSameDT=off  OutDataTypeStr=boolean
  Memory : Memory  InheritSampleTime=on
  Saturation : Saturate  UpperLimit=200  LowerLimit=-1
      settings: AttributesFormatString="Min = %<LowerLimit>  Max = %<UpperLimit>"
  Switch : Switch  Criteria=u2 > Threshold
  EmgcyLghtEC_stEmgcyLghtECFlg : Outport
  wires:
  Compare To Constant3/1 -> Logical Operator/3
  Bus Selector/3 -> Compare To Constant3/1  "<BCM_Right_Light>"
  Compare To Constant/1 -> EmgcyLghtEC_stEmgcyLghtECFlg/1
  Memory/1 -> Add/2
  Saturation/1 -> Memory/1, Compare To Constant/1
  Add/1 -> Saturation/1
  Switch/1 -> Add/1
  Constant1/1 -> Switch/3
  Constant/1 -> Switch/1
  Logical Operator/1 -> Switch/2
  Bus Selector/2 -> Compare To Constant2/1  "<BCM_Left_Light>"
  Bus Selector/1 -> Compare To Constant1/1  "<BCM_Double_Light>"
  EmgcyLghtEC_bsStLampState/1 -> Bus Selector/1
  Compare To Constant1/1 -> Logical Operator/1
  Compare To Constant2/1 -> Logical Operator/2

== system LKAS_AutoSave_DF_20211126_SW5/LKAS/LL/LLOn/LL State Determination (LLStateDet)/LL State Machine Conditions (LLSMCon)/Enable Condition (EnaC)/Vehicle State Condition (VehStateC)/Gear Enable Condition (GearEC) ==
  GearEC_bsTCUState : Inport
  Bus Selector : BusSelector  OutputSignals=TCU_ActualGear
  Compare To Constant : simulink/Logic and Bit Operations/Compare To Constant  relop===  const=3  OutDataTypeStr=boolean
  GearEC_stGearECFlg : Outport
  wires:
  Compare To Constant/1 -> GearEC_stGearECFlg/1
  Bus Selector/1 -> Compare To Constant/1  "<TCU_ActualGear>"
  GearEC_bsTCUState/1 -> Bus Selector/1

== system LKAS_AutoSave_DF_20211126_SW5/LKAS/LL/LLOn/LL State Determination (LLStateDet)/LL State Machine Conditions (LLSMCon)/Enable Condition (EnaC)/Vehicle State Condition (VehStateC)/Vehicle Speed Enable Condition (VehSpdEC) ==
  VehSpdEC_stDACMode : Inport
  VehSpdEC_vVehSpd : Inport  Port=2
  VehSpdEC_vLDWVehSpdMax_C : Inport  Port=3
  VehSpdEC_vLKAVehSpdMax_C : Inport  Port=4
  VehSpdEC_vVehSpdMin_C : Inport  Port=5
  Interval Test Dynamic : simulink/Logic and Bit Operations/Interval Test Dynamic  IntervalClosedRight=on  IntervalClosedLeft=on  OutDataTypeStr=boolean
      settings: SourceProductName=Simulink  SourceProductBaseCode=SL
  Switch : Switch  Threshold=2
  VehSpdEC_stVehSpdECFlg : Outport
  wires:
  VehSpdEC_vLDWVehSpdMax_C/1 -> Switch/3
  Switch/1 -> Interval Test Dynamic/1
  VehSpdEC_vLKAVehSpdMax_C/1 -> Switch/1
  VehSpdEC_stDACMode/1 -> Switch/2
  Interval Test Dynamic/1 -> VehSpdEC_stVehSpdECFlg/1
  VehSpdEC_vVehSpdMin_C/1 -> Interval Test Dynamic/3
  VehSpdEC_vVehSpd/1 -> Interval Test Dynamic/2

== system LKAS_AutoSave_DF_20211126_SW5/LKAS/LL/LLOn/LL State Determination (LLStateDet)/LL State Machine Conditions (LLSMCon)/Enable Condition (EnaC)/Vehicle State Condition (VehStateC)/Vehicle State Condition Synthesis (VehStateCSyn) ==
  VehStateCSyn_stVehSpdECFlg : Inport
  VehStateCSyn_stEmgcyLghtECFlg : Inport  Port=2
  VehStateCSyn_stGearECFlg : Inport  Port=3
  Logical Operator : Logic  Inputs=3  AllPortsSameDT=off  OutDataTypeStr=boolean
  VehStateCSyn_stVehStateCSyn : Outport
  wires:
  VehStateCSyn_stEmgcyLghtECFlg/1 -> Logical Operator/2
  Logical Operator/1 -> VehStateCSyn_stVehStateCSyn/1
  VehStateCSyn_stGearECFlg/1 -> Logical Operator/3
  VehStateCSyn_stVehSpdECFlg/1 -> Logical Operator/1

== system LKAS_AutoSave_DF_20211126_SW5/LKAS/LL/LLOn/LKA/LKA Motion Planning (LKAMP) /Switching Condition (SwtCon)/Ending Heading Angle Determination (EndHdAgDet)/Lateral Speed Compensation (LSpdComp)/If Action Subsystem ==
  In1 : Inport
  Action Port : ActionPort  InitializeStates=reset  ActionType=then
      settings: AttributesFormatString=states = %<InitializeStates>
  Cast To Single1 : DataTypeConversion  LockScale=on
  Out1 : Outport  InitialOutput=0
      settings: AttributesFormatString=%<OutputWhenDisabled> = %<InitialOutput>
  wires:
  In1/1 -> Cast To Single1/1
  Cast To Single1/1 -> Out1/1

== system LKAS_AutoSave_DF_20211126_SW5/LKAS/LL/LLOn/LKA/LKA Motion Planning (LKAMP) /Switching Condition (SwtCon)/Ending Heading Angle Determination (EndHdAgDet)/Lateral Speed Compensation (LSpdComp)/If Action Subsystem2 ==
  Action Port : ActionPort  InitializeStates=reset  ActionType=else
      settings: AttributesFormatString=states = %<InitializeStates>
  Constant : Constant  Value=0  OutDataTypeStr=single
  Out1 : Outport  InitialOutput=0
      settings: AttributesFormatString=%<OutputWhenDisabled> = %<InitialOutput>
  wires:
  Constant/1 -> Out1/1

== system LKAS_AutoSave_DF_20211126_SW5/LKAS/LL/LLOn/LKA/LKA Motion Planning (LKAMP) /Switching Condition (SwtCon)/Ending Heading Angle Determination (EndHdAgDet)/Lateral Speed Compensation (LSpdComp)/If Action Subsystem4 ==
  In1 : Inport
  Action Port : ActionPort  InitializeStates=reset  ActionType=elseif
      settings: AttributesFormatString=states = %<InitializeStates>
  Cast To Single1 : DataTypeConversion  LockScale=on
  Out1 : Outport  InitialOutput=0
      settings: AttributesFormatString=%<OutputWhenDisabled> = %<InitialOutput>
  wires:
  In1/1 -> Cast To Single1/1
  Cast To Single1/1 -> Out1/1

== system LKAS_AutoSave_DF_20211126_SW5/LKAS/LL/LLOn/LKA/Lane Following (LF)/Trajectory Following Control (TFC)/Feedback Control (FbCtl)/Subsystem/If Action Subsystem ==
  In1 : Inport
  Action Port : ActionPort  ActionType=then
      settings: AttributesFormatString=states = %<InitializeStates>
  Out1 : Outport
      settings: AttributesFormatString=%<OutputWhenDisabled> = %<InitialOutput>
  wires:
  In1/1 -> Out1/1

== system LKAS_AutoSave_DF_20211126_SW5/LKAS/LL/LLOn/LKA/Lane Following (LF)/Trajectory Following Control (TFC)/Feedback Control (FbCtl)/Subsystem/If Action Subsystem1 ==
  In1 : Inport
  Action Port : ActionPort  ActionType=elseif
      settings: AttributesFormatString=states = %<InitializeStates>
  Out1 : Outport
      settings: AttributesFormatString=%<OutputWhenDisabled> = %<InitialOutput>
  wires:
  In1/1 -> Out1/1

== system LKAS_AutoSave_DF_20211126_SW5/LKAS/LL/LLOn/LKA/Lane Following (LF)/Trajectory Following Control (TFC)/Feedback Control (FbCtl)/Subsystem/If Action Subsystem2 ==
  In1 : Inport
  Action Port : ActionPort  ActionType=else
      settings: AttributesFormatString=states = %<InitializeStates>
  Out1 : Outport
      settings: AttributesFormatString=%<OutputWhenDisabled> = %<InitialOutput>
  wires:
  In1/1 -> Out1/1

== system LKAS_AutoSave_DF_20211126_SW5/LKAS/LL/LLOn/LKA/Lane Following (LF)/Trajectory Following Control (TFC)/Feedback Control (FbCtl)/Subsystem/Signal Latching2 ==
  In : Inport
  Add : Sum  OutDataTypeStr=uint16
  Constant : Constant  OutDataTypeStr=uint16  SampleTime=-1
  Constant2 : Constant  Value=LatchTime  OutDataTypeStr=uint16  SampleTime=-1
  If : If  NumInputs=2  IfExpression=u1==u2  ShowElse=off
  Memory : Memory  InheritSampleTime=on
  Saturation1 : Saturate  UpperLimit=10000  LowerLimit=0  OutDataTypeStr=uint16
  "if action " : Subsystem  TreatAsAtomicUnit=on
  Out : Outport
  wires:
  Saturation1/1 -> If/1, Memory/1
  Memory/1 -> Add/2
  Add/1 -> Saturation1/1
  Constant/1 -> Add/1
  If/1 -> "if action "/Action
  "if action "/1(Out) -> Out/1
  In/1 -> "if action "/1(In)
  Constant2/1 -> If/2

== system LKAS_AutoSave_DF_20211126_SW5/LKAS/LL/LLOn/LKA/Plan To LaneFollowing (PTLF)/InsideJudge1/If Action Subsystem/If Action Subsystem/Signal Latching ==
  In : Inport
  Add : Sum  OutDataTypeStr=uint16
  Constant : Constant  OutDataTypeStr=uint16  SampleTime=-1
  Constant2 : Constant  Value=LatchTime  OutDataTypeStr=uint16  SampleTime=-1
  If : If  NumInputs=2  IfExpression=u1<=u2  ShowElse=off
  Memory : Memory  InheritSampleTime=on
  Saturation1 : Saturate  UpperLimit=10000  LowerLimit=0  OutDataTypeStr=uint16
  "if action " : Subsystem  TreatAsAtomicUnit=on
  Out : Outport
  wires:
  Constant2/1 -> If/2
  In/1 -> "if action "/1(In)
  "if action "/1(Out) -> Out/1
  If/1 -> "if action "/Action
  Constant/1 -> Add/1
  Add/1 -> Saturation1/1
  Memory/1 -> Add/2
  Saturation1/1 -> Memory/1, If/1
